simulink model "RobotskiManipulator"  (R2015b)
settings: Solver=ode45  StartTime=0.0  StopTime=40  RelTol=1e-3
undefined symbols (not defined in the file or in its folder): a1, a2, g, m1, m2
settings Model: Creator=Inspiron  LastModifiedBy=user
settings DataIOCC: SaveFormat=Array
settings OptimizationCC: ExpressionDepthLimit=2147483647
settings DebuggingCC: UnderspecifiedInitializationDetection=Classic  MergeDetectMultiDrivingBlocksExec=none  SolverPrmCheckMsg=warning  StateNameClashWarn=warning
settings HardwareCC: ProdBitPerPointer=32  ProdLargestAtomicFloat=None  ProdIntDivRoundTo=Undefined  ProdEndianess=Unspecified  ProdWordSize=32  ProdHWDeviceType=32-bit Generic
settings GRTTargetCC: GeneratePreprocessorConditionals=Disable all
settings ConfigComp: CovModelRefEnable=Off

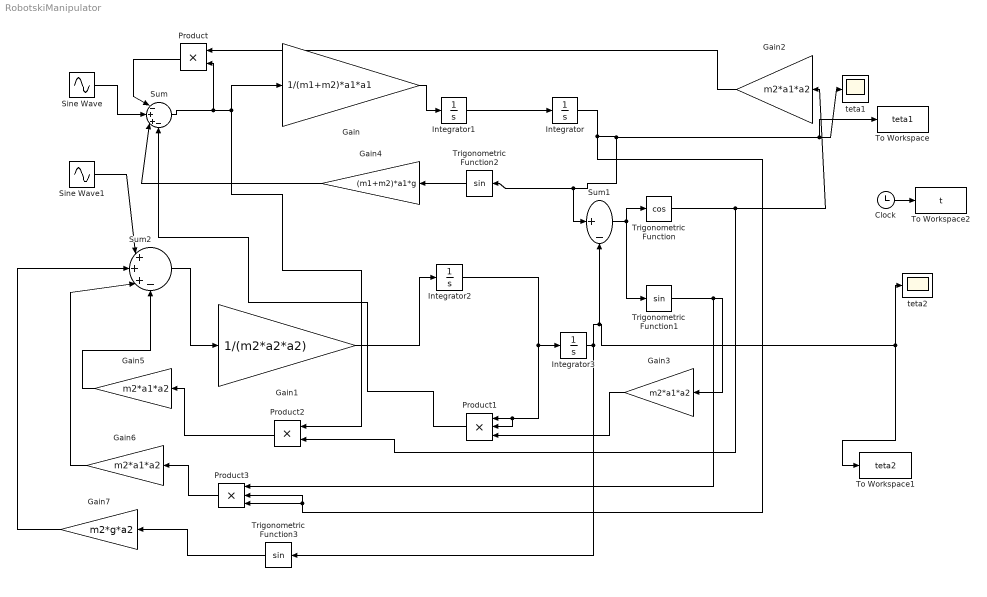
== system RobotskiManipulator ==
  Clock : Clock
  Gain : Gain  Gain=1/(m1+m2)*a1*a1
  Gain1 : Gain  Gain=1/(m2*a2*a2)
  Gain{2..3,5..6} (4 alike) : Gain  Gain=m2*a1*a2
  Gain4 : Gain  Gain=(m1+m2)*a1*g
  Gain7 : Gain  Gain=m2*g*a2
  Integrator{,1..3} (4 alike) : Integrator
  Product : Product  RndMeth=Zero
  Product1 : Product  Inputs=3  RndMeth=Zero
  Product2 : Product  RndMeth=Zero
  Product3 : Product  Inputs=3  RndMeth=Zero
  Sine Wave : Sin  Amplitude=3  Frequency=2  SampleTime=0
  Sine Wave1 : Sin  Amplitude=3  Frequency=4  SampleTime=0
  Sum : Sum  Inputs=|-++-
  Sum1 : Sum  Inputs=|+-
  Sum2 : Sum  Inputs=|+++-
  To Workspace : ToWorkspace  VariableName=teta1  SampleTime=-1
      settings: Save2DSignal=2-D array (concatenate along first dimension)
  To Workspace1 : ToWorkspace  VariableName=teta2  SampleTime=-1
      settings: Save2DSignal=2-D array (concatenate along first dimension)
  To Workspace2 : ToWorkspace  VariableName=t  SampleTime=-1
      settings: Save2DSignal=2-D array (concatenate along first dimension)
  Trigonometric Function : Trigonometry  Operator=cos
  Trigonometric Function1 : Trigonometry
  Trigonometric Function2 : Trigonometry
  Trigonometric Function3 : Trigonometry
  teta1 : Scope
  teta2 : Scope
  wires:
  Sum/1 -> Product2/1, Gain/1, Product/2
  Gain/1 -> Integrator1/1
  Integrator1/1 -> Integrator/1
  Integrator/1 -> Product3/3, Product3/2, teta1/1, To Workspace/1, Trigonometric Function2/1, Sum1/1
  Sum1/1 -> Trigonometric Function/1, Trigonometric Function1/1
  Sum2/1 -> Gain1/1
  Gain1/1 -> Integrator2/1
  Integrator2/1 -> Product1/2, Product1/1, Integrator3/1
  Integrator3/1 -> teta2/1, To Workspace1/1, Sum1/2, Trigonometric Function3/1
  Trigonometric Function/1 -> Gain2/1, Product2/2
  Gain2/1 -> Product/1
  Product/1 -> Sum/1
  Trigonometric Function1/1 -> Product3/1, Gain3/1
  Gain3/1 -> Product1/3
  Product1/1 -> Sum/4
  Trigonometric Function2/1 -> Gain4/1
  Gain4/1 -> Sum/3
  Product2/1 -> Gain5/1
  Gain5/1 -> Sum2/4
  Product3/1 -> Gain6/1
  Gain6/1 -> Sum2/3
  Trigonometric Function3/1 -> Gain7/1
  Gain7/1 -> Sum2/2
  Clock/1 -> To Workspace2/1
  Sine Wave/1 -> Sum/2
  Sine Wave1/1 -> Sum2/1
